simulink model "SCR_SiLS_R4"  (R2023a)
settings: Solver=VariableStepAuto  StartTime=0.0  StopTime=T_sim_end  RelTol=1e-3
model workspace (MAT data in the model file):
  ConnVar.ipAddress = '192.168.0.153'
  ConnVar.user = 'M1'
  ConnVar.pwd = [145 145 158 146 151 156 158 157]
  ConnVar.targetHandle = 0
libraries: simulink x4, M1SWBlocks x4
settings Model: Creator=CHSE  LastModifiedBy=gione
settings DebuggingCC: UnconnectedInputMsg=warning  UnconnectedOutputMsg=warning  UnconnectedLineMsg=warning
settings ModelReferenceCC: EnableRefExpFcnMdlSchedulingChecks=on
settings RTWCC: DLArmComputeVersion=19.05

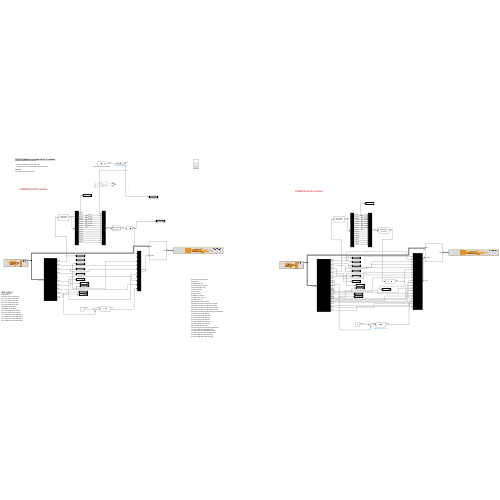
[thumbnail: Simulink's stored preview of the top-level diagram]
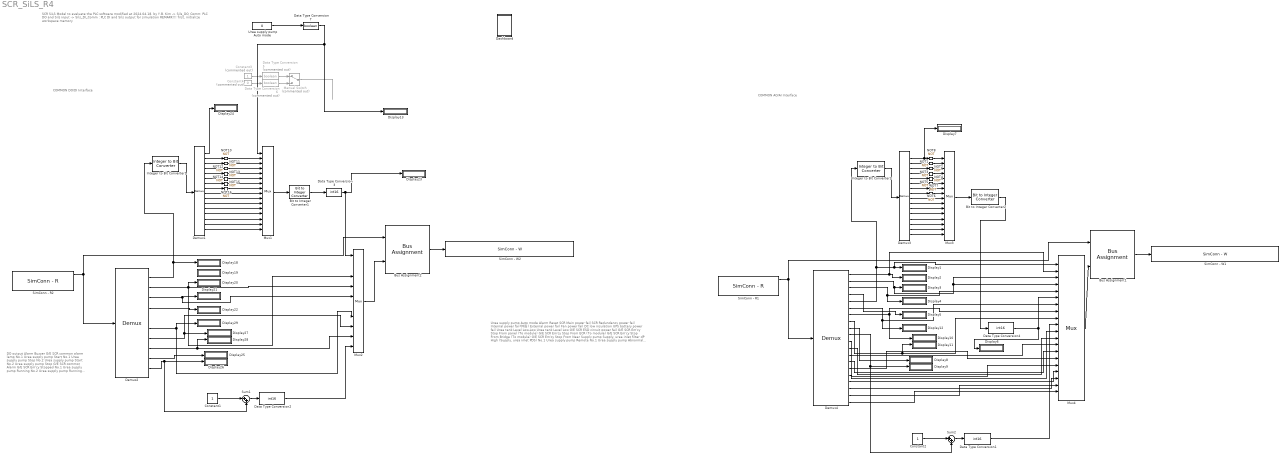
== system SCR_SiLS_R4 ==
  note: DO output
      | Alarm Buzzer
      |
      | G/E SCR common alarm lamp
      |
      | No.1 Urea supply pump Start
      |
      | No.1 Urea supply pump Stop
      |
      | No.2 Urea supply pump Start
      |
      | No.2 Urea supply pump Stop
      |
      | G/E SCR common Alarm
      |
      | G/E SCR Em'cy Stopped
      |
      | No.1 Urea supply pump Running
      |
      | No.2 Urea supply pump Running
      |
      | No.1 G/E SCR Common Alarm lamp
      |
      | No.2 G/E SCR Common Alarm lamp
      |
      | No.3 G/E SCR Common Alarm lamp
      |
      | No.4 G/E SCR Common Alarm lamp
      |
      | ​
      |
      | ​
  note: Urea supply pump Auto mode
      |
      | Alarm Reset
      |
      | SCR Main power fail
      |
      | SCR Redundancy power fail
      |
      | Internal power fail(삭제됨)
      |
      | External power fail
      |
      | Fan power fail
      |
      | DC low insulation
      |
      | UPS battery power fail
      |
      | Urea tank Level Low-Low
      |
      | Urea tank Level Low
      |
      | G/E SCR ESD circuit power fail
      |
      | G/E SCR Em'cy Stop From panel (To module)
      |
      | G/E SCR Em'cy Stop From ECR (To module)
      |
      | G/E SCR Em'cy Stop From Bridge (To module)
      |
      | G/E SCR Em'cy Stop From Near Supply pump
      |
      | Supply, urea inlet filter dP High (Supply, urea inlet PDS)
      |
      | No.1 Urea supply pump Remote
      |
      | No.1 Urea supply pump Abnormal
      |
      | No.1 Urea supply pump Running
      |
      | No.2 Urea supply pump Remote
      |
      | No.2 Urea supply pump Abnormal
      |
      | No.2 Urea supply pump Running
      |
      | G/E Low Sulfur fuel supplied
      |
      | Urea tank drip tray Level High-High (ABS class)
      |
      | Urea tank TEMP High-High (ABS class)
      |
      | Urea tank Level High (ABS, BV, NK class)
      |
      | Urea tank drip tray Level High (ABS class)
      |
      | Urea tank TEMP Low (ABS, NK class)
      |
      | Urea tank TEMP High (ABS, NK class)
      |
      | ​
      |
      | ​
  note: COMMON DO/DI Interface
  note: SCR SiLS Model to evaluate the PLC software
      | modified at 2024.04.18. by Y.B. Kim
      |
      | -> Sils_DO_Comm: PLC DO and Sils input
      | -> Sils_DI_Comm : PLC DI and Sils output for simulation
      |
      | REMARK!!!
      | first, initialize workspace memory
  note: COMMON AO/AI Interface
  Bit to Integer Converter1 : simulink/Logic and Bit Operations/Bit to Integer Converter  nbits=16  bitOrder=LSB first  signedOutputValues=Unsigned  outDtype=Inherit via internal rule  outDtypeSigned=Inherit via internal rule
  Bit to Integer Converter2 : simulink/Logic and Bit Operations/Bit to Integer Converter  nbits=16  bitOrder=LSB first  signedOutputValues=Unsigned  outDtype=Inherit via internal rule  outDtypeSigned=Inherit via internal rule
  Bus Assignment1 : BusAssignment  AssignedSignals=data
  Bus Assignment2 : BusAssignment  AssignedSignals=data
  Constant1 : Constant
  Constant2 : Constant
  Constant3 : Constant  Commented=on  OutDataTypeStr=boolean
  Constant4 : Constant  Commented=on  Value=0  OutDataTypeStr=boolean
  Dashboard : Subsystem
  Data Type Conversion{1..4} (4 alike) : DataTypeConversion  OutDataTypeStr=int16  SaturateOnIntegerOverflow=off  RndMeth=Floor
  Data Type Conversion5 : DataTypeConversion  Commented=on  OutDataTypeStr=boolean  SaturateOnIntegerOverflow=off  RndMeth=Floor
  Data Type Conversion6 : DataTypeConversion  Commented=on  OutDataTypeStr=boolean  SaturateOnIntegerOverflow=off  RndMeth=Floor
  Data Type Conversion7 : DataTypeConversion  OutDataTypeStr=boolean  SaturateOnIntegerOverflow=off  RndMeth=Floor
  Demux1 : Demux  Outputs=16
  Demux2 : Demux  Outputs=10
  Demux3 : Demux  Outputs=16
  Demux4 : Demux  Outputs=20
  Display{1..13,18..29} (25 alike) : Display
      Display20 settings: Format=decimal (Stored Integer)
      Display3 settings: Format=decimal (Stored Integer)
  Integer to Bit Converter1 : simulink/Logic and Bit Operations/Integer to Bit Converter  nbits=16  signedInputValues=Unsigned  bitOrder=LSB first  outDtype=boolean
  Integer to Bit Converter2 : simulink/Logic and Bit Operations/Integer to Bit Converter  nbits=16  signedInputValues=Unsigned  bitOrder=LSB first  outDtype=boolean
  Manual Switch : ManualSwitch  Commented=on
  Mux1 : Mux  Inputs=16
  Mux2 : Mux  Inputs=10
  Mux3 : Mux  Inputs=16
  Mux4 : Mux  Inputs=20
  NOT{1..8,10..16} (15 alike) : Logic  Operator=NOT  IconShape=distinctive  AllPortsSameDT=off  OutDataTypeStr=boolean
  SimConn - R1 : M1SWBlocks/SimConn Blocks/SimConn - R  connVarName=ConnVar  InswModuleName='NONOXR4'  swModuleName=NONOXR4  InvarName='.Sils_AO_Comm'  varName=.Sils_AO_Comm  varDataType=Bus: IOSim_AIO_typ  enRetOutput=on  enGetTrigger=off  getTrigger=rising  valDurLostConn=Zero  internalVal=0  DataDim=1  enSampTimMon=on  sampleTime=Ts_com
      settings: SourceProductName=Bachmann M1 Software
  SimConn - R2 : M1SWBlocks/SimConn Blocks/SimConn - R  connVarName=ConnVar  InswModuleName='NONOXR4'  swModuleName=NONOXR4  InvarName='.Sils_DO_Comm'  varName=.Sils_DO_Comm  varDataType=Bus: IOSim_typ  enRetOutput=on  enGetTrigger=off  getTrigger=rising  valDurLostConn=Zero  internalVal=0  DataDim=1  enSampTimMon=on  sampleTime=Ts_com
      settings: SourceProductName=Bachmann M1 Software
  SimConn - W1 : M1SWBlocks/SimConn Blocks/SimConn - W  connVarName=ConnVar  InswModuleName='NONOXR4'  swModuleName=NONOXR4  InvarName='.Sils_AI_Comm'  varName=.Sils_AI_Comm  varDataType=Bus: IOSim_AIO_typ  enRetOutput=off  enGetTrigger=off  getTrigger=rising  enSampTimMon=off
      settings: SourceProductName=Bachmann M1 Software
  SimConn - W2 : M1SWBlocks/SimConn Blocks/SimConn - W  connVarName=ConnVar  InswModuleName='NONOXR4'  swModuleName=NONOXR4  InvarName='.Sils_DI_Comm'  varName=.Sils_DI_Comm  varDataType=Bus: IOSim_typ  enRetOutput=off  enGetTrigger=off  getTrigger=rising  enSampTimMon=off
      settings: SourceProductName=Bachmann M1 Software
  Sum1 : Sum  Inputs=|++
  Sum2 : Sum  Inputs=|++
  Urea supply pump Auto mode : Constant  Value=0
  wires:
  Demux1/7 -> NOT15/1
  Demux1/2 -> NOT10/1
  NOT16/1 -> Mux1/8
  Demux1/6 -> NOT14/1
  Demux1/12 -> Mux1/12
  NOT10/1 -> Mux1/2
  Demux1/13 -> Mux1/13
  NOT13/1 -> Mux1/5
  Demux1/9 -> Mux1/9
  Integer to Bit Converter1/1 -> Demux1/1
  Demux1/14 -> Mux1/14
  Mux1/1 -> Bit to Integer Converter1/1
  Bit to Integer Converter1/1 -> Data Type Conversion3/1
  Demux1/4 -> NOT12/1
  Demux1/16 -> Mux1/16
  Demux1/11 -> Mux1/11
  Demux1/10 -> Mux1/10
  NOT14/1 -> Mux1/6
  Demux2/3 -> Mux2/5, Display21/1
  Data Type Conversion3/1 -> Display23/1, Mux2/1
  NOT12/1 -> Mux1/4
  Demux1/3 -> NOT11/1
  Constant1/1 -> Sum1/1
  Demux2/4 -> Display22/1
  Sum1/1 -> Data Type Conversion2/1
  Demux2/2 -> Display20/1, Mux2/3, Mux2/4
  NOT11/1 -> Mux1/3
  Demux1/5 -> NOT13/1
  NOT15/1 -> Mux1/7
  Demux1/15 -> Mux1/15
  Demux1/8 -> NOT16/1
  SimConn - R2/1 -> Bus Assignment2/1, Demux2/1
  Demux2/9 -> Display25/1
  Demux2/10 -> Sum1/2, Display26/1
  Demux2/8 -> Mux2/9, Display28/1
  Demux2/7 -> Mux2/8, Display27/1
  Demux2/6 -> Mux2/7, Display29/1
  Mux2/1 -> Bus Assignment2/2
  Bus Assignment2/1 -> SimConn - W2/1
  Data Type Conversion2/1 -> Mux2/10
  Demux4/6 -> Display12/1, Mux4/7
  Bus Assignment1/1 -> SimConn - W1/1
  Demux4/9 -> Display8/1
  Demux4/7 -> Display10/1, Mux4/8
  Mux4/1 -> Bus Assignment1/2
  Demux4/10 -> Sum2/2, Display9/1
  Demux4/1 -> Mux4/2, Display2/1
  Data Type Conversion1/1 -> Mux4/10
  Demux4/8 -> Mux4/9, Display11/1
  Demux3/8 -> NOT7/1
  Demux4/5 -> Integer to Bit Converter2/1, Mux4/1, Display1/1
  Demux3/15 -> Mux3/15
  NOT6/1 -> Mux3/7
  Data Type Conversion4/1 -> Mux4/6, Display6/1
  NOT1/1 -> Mux3/2
  SimConn - R1/1 -> Bus Assignment1/1, Demux4/1
  Demux3/7 -> NOT6/1
  Demux3/1 -> Display7/1, NOT8/1
  Demux4/4 -> Display5/1
  Demux3/5 -> NOT4/1
  NOT5/1 -> Mux3/6
  Integer to Bit Converter2/1 -> Demux3/1
  Demux3/3 -> NOT2/1
  Demux3/4 -> NOT3/1
  Demux4/2 -> Mux4/3, Mux4/4, Display3/1
  NOT3/1 -> Mux3/4
  Demux3/9 -> Mux3/9
  Sum2/1 -> Data Type Conversion1/1
  Demux3/11 -> Mux3/11
  Demux3/13 -> Mux3/13
  Demux3/16 -> Mux3/16
  Constant2/1 -> Sum2/1
  NOT8/1 -> Mux3/1
  NOT4/1 -> Mux3/5
  Demux4/3 -> Display4/1, Mux4/5
  Demux3/14 -> Mux3/14
  Mux3/1 -> Bit to Integer Converter2/1
  Demux3/10 -> Mux3/10
  Demux3/2 -> NOT1/1
  Demux3/6 -> NOT5/1
  NOT7/1 -> Mux3/8
  Demux3/12 -> Mux3/12
  Bit to Integer Converter2/1 -> Data Type Conversion4/1
  NOT2/1 -> Mux3/3
  Demux4/11 -> Mux4/11
  Demux4/12 -> Mux4/12
  Demux4/13 -> Mux4/13
  Demux4/14 -> Mux4/14
  Demux4/15 -> Mux4/15
  Demux4/16 -> Mux4/16
  Demux4/17 -> Mux4/17
  Demux4/18 -> Mux4/18
  Demux4/19 -> Mux4/19
  Demux4/20 -> Mux4/20
  Demux2/1 -> Integer to Bit Converter1/1, Display18/1
  Demux1/1 -> Display24/1
  Constant3/1 -> Data Type Conversion5/1
  Constant4/1 -> Data Type Conversion6/1
  Manual Switch/1 -> ?
  Data Type Conversion5/1 -> Manual Switch/1
  Data Type Conversion6/1 -> Manual Switch/2
  Urea supply pump Auto mode/1 -> Data Type Conversion7/1
  Data Type Conversion7/1 -> Display13/1, Mux1/1

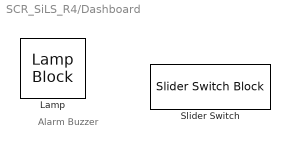
== system SCR_SiLS_R4/Dashboard ==
  note: Alarm Buzzer
  Lamp : LampBlock  LabelPosition=Hide
  Slider Switch : SliderSwitchBlock
      settings: Values={{'Off', 'On'}, [0 1]}
